simulink model "brake_in_car"  (R2024b)
settings: Solver=VariableStepAuto  StartTime=0.0  StopTime=inf  RelTol=1e-3
values from neighbouring files (symbols this model uses):
  A = 2    [evin_parameters.m]    (also in parameters.m)
  c_1 = 0.86    [evin_parameters.m]    (also in parameters.m)
  c_2 = 33.82    [evin_parameters.m]    (also in parameters.m)
  c_3 = 0.36    [evin_parameters.m]    (also in parameters.m)
  cw = 0.3    [parameters.m]
  g = 9.81    [evin_parameters.m]    (also in parameters.m)
  J = 0.8    [parameters.m]
  m = 1500    [evin_parameters.m]    (also in parameters.m)
  r = 0.3    [parameters.m]
  rho = 1.2    [evin_parameters.m]    (also in parameters.m)
  T_w = 5355    [parameters.m]
  x1 = 0    [parameters.m]
  x2 = 100    [parameters.m]
libraries: simulink x2
settings Model: Creator=kavin  LastModifiedBy=kavin
settings SolverCC: ZeroCrossAlgorithm=Adaptive
settings DebuggingCC: IgnoredZcDiagnostic=none

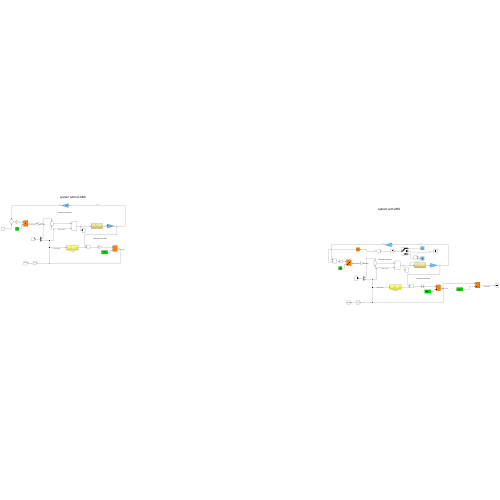
[thumbnail: Simulink's stored preview of the top-level diagram]
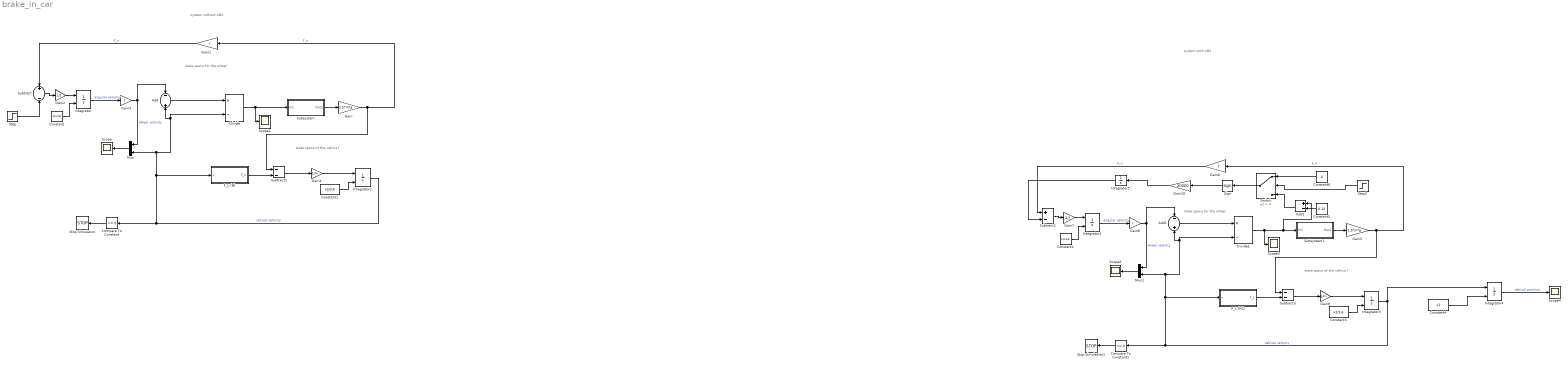
== system brake_in_car ==
  note: system without ABS
  note: state space of the vehica l
  note: state space for the wheel
  note: state space for the wheel
  note: state space of the vehica l
  note: system with ABS
  Add : Sum  Inputs=-+
  Add1 : Sum  Inputs=-+
  Add2 : Sum  Inputs=+-
  Compare To Constant : simulink/Logic and Bit Operations/Compare To Constant  relop=<=  const=0  OutDataTypeStr=boolean
  Compare To Constant1 : simulink/Logic and Bit Operations/Compare To Constant  relop=<=  const=0  OutDataTypeStr=boolean
  Constant : Constant  Value=x2/(r*3)
  Constant1 : Constant  Value=x2/3.6
  Constant2 : Constant  Value=x2/r/3.6
  Constant3 : Constant  Value=x2/3.6
  Constant4 : Constant  Value=x1
  Constant5 : Constant  Value=0.13
  Constant6 : Constant  Value=0
  Divide : Product  Inputs=*/
  Divide1 : Product  Inputs=*/
  F_L (N) : Subsystem
  F_L (N)1 : Subsystem
  Gain : Gain  Gain=1.5*m*g
  Gain{1,3,6,8} (4 alike) : Gain  Gain=r
  Gain10 : Gain  Gain=20000
  Gain2 : Gain  Gain=1/J
  Gain4 : Gain  Gain=1/m
  Gain5 : Gain  Gain=1.5*m*g
  Gain7 : Gain  Gain=1/J
  Gain9 : Gain  Gain=1/m
  Integrator : Integrator  InitialConditionSource=external
  Integrator1 : Integrator  InitialConditionSource=external  LimitOutput=on  LowerSaturationLimit=0
  Integrator2 : Integrator  InitialConditionSource=external
  Integrator3 : Integrator  InitialConditionSource=external  LimitOutput=on  LowerSaturationLimit=0
  Integrator4 : Integrator  InitialConditionSource=external  LimitOutput=on  LowerSaturationLimit=0
  Integrator5 : Integrator  LimitOutput=on  LowerSaturationLimit=0
  Mux : Mux  Inputs=2
  Mux1 : Mux  Inputs=2
  Scope{,1..4} (5 alike) : Scope
  Sign : Signum
  Step : Step  After=T_w  SampleTime=0
  Step2 : Step  SampleTime=0
  Stop Simulation : Stop
  Stop Simulation1 : Stop
  Subsystem : Subsystem
  Subsystem1 : Subsystem
  Subtract : Sum  Inputs=+-
  Subtract1 : Sum  Inputs=--
  Subtract2 : Sum  Inputs=+-
  Subtract3 : Sum  Inputs=--
  Switch : Switch  Criteria=u2 > Threshold  SaturateOnIntegerOverflow=off  InputSameDT=off
  wires:
  Subsystem/1(Out1) -> Gain/1
  Gain/1 -> Gain1/1, Subtract1/1  "F_n"
  Gain1/1 -> Subtract/1  "F_n"
  Step/1 -> Subtract/2
  Gain2/1 -> Integrator/1
  Subtract/1 -> Gain2/1
  Constant/1 -> Integrator/2
  Integrator/1 -> Gain3/1  "angular velocity"
  Gain3/1 -> Mux/1, Add/1  "wheel velocity"
  F_L (N)/1(F_L) -> Subtract1/2
  Subtract1/1 -> Gain4/1
  Gain4/1 -> Integrator2/1
  Integrator2/1 -> Compare To Constant/1, Divide/2, Add/2, Mux/2, F_L (N)/1(v)  "vehical velocity"
  Constant1/1 -> Integrator2/2
  Compare To Constant/1 -> Stop Simulation/1
  Mux/1 -> Scope/1
  Add/1 -> Divide/1
  Divide/1 -> Scope1/1, Subsystem/1(In1)
  Divide1/1 -> Scope3/1, Add2/2, Subsystem1/1(In1)
  Add1/1 -> Divide1/1
  Subtract2/1 -> Gain7/1
  Gain9/1 -> Integrator3/1
  Gain7/1 -> Integrator1/1
  Constant2/1 -> Integrator1/2
  Compare To Constant1/1 -> Stop Simulation1/1
  F_L (N)1/1(F_L) -> Subtract3/2
  Gain8/1 -> Mux1/1, Add1/1  "wheel velocity"
  Subtract3/1 -> Gain9/1
  Gain6/1 -> Subtract2/1  "F_n"
  Integrator3/1 -> Compare To Constant1/1, Divide1/2, Add1/2, Mux1/2, F_L (N)1/1(v), Integrator4/1  "vehical velocity"
  Subsystem1/1(Out1) -> Gain5/1
  Integrator1/1 -> Gain8/1  "angular velocity"
  Gain5/1 -> Gain6/1, Subtract3/1  "F_n"
  Mux1/1 -> Scope2/1
  Constant3/1 -> Integrator3/2
  Constant4/1 -> Integrator4/2
  Integrator4/1 -> Scope4/1  "vehical position"
  Add2/1 -> Switch/3
  Constant5/1 -> Add2/1
  Step2/1 -> Switch/2
  Switch/1 -> Sign/1
  Constant6/1 -> Switch/1
  Sign/1 -> Gain10/1
  Gain10/1 -> Integrator5/1
  Integrator5/1 -> Subtract2/2

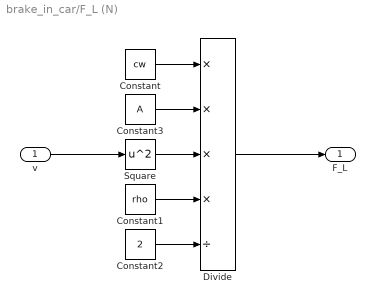
== system brake_in_car/F_L (N) ==
  v : Inport
  Constant : Constant  Value=cw
  Constant1 : Constant  Value=rho
  Constant2 : Constant  Value=2
  Constant3 : Constant  Value=A
  Divide : Product  Inputs=****/
  Square : Math  Operator=square
  F_L : Outport
  wires:
  v/1 -> Square/1
  Divide/1 -> F_L/1
  Square/1 -> Divide/3
  Constant2/1 -> Divide/5
  Constant/1 -> Divide/1
  Constant3/1 -> Divide/2
  Constant1/1 -> Divide/4

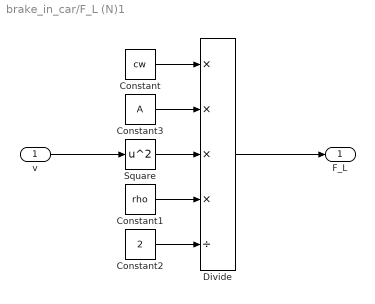
== system brake_in_car/F_L (N)1 ==
  v : Inport
  Constant : Constant  Value=cw
  Constant1 : Constant  Value=rho
  Constant2 : Constant  Value=2
  Constant3 : Constant  Value=A
  Divide : Product  Inputs=****/
  Square : Math  Operator=square
  F_L : Outport
  wires:
  v/1 -> Square/1
  Divide/1 -> F_L/1
  Square/1 -> Divide/3
  Constant2/1 -> Divide/5
  Constant/1 -> Divide/1
  Constant3/1 -> Divide/2
  Constant1/1 -> Divide/4

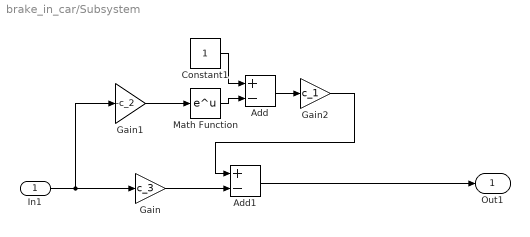
== system brake_in_car/Subsystem ==
  In1 : Inport
      settings: AttributesFormatString=|
      | %<BlockType>
      | lambda
  Add : Sum  Inputs=+-
  Add1 : Sum  Inputs=+-
  Constant1 : Constant
  Gain : Gain  Gain=c_3
  Gain1 : Gain  Gain=-c_2
  Gain2 : Gain  Gain=c_1
  Math Function : Math
  Out1 : Outport
      settings: AttributesFormatString=mu
  wires:
  In1/1 -> Gain1/1, Gain/1
  Gain1/1 -> Math Function/1
  Math Function/1 -> Add/2
  Constant1/1 -> Add/1
  Add/1 -> Gain2/1
  Gain2/1 -> Add1/1
  Add1/1 -> Out1/1
  Gain/1 -> Add1/2

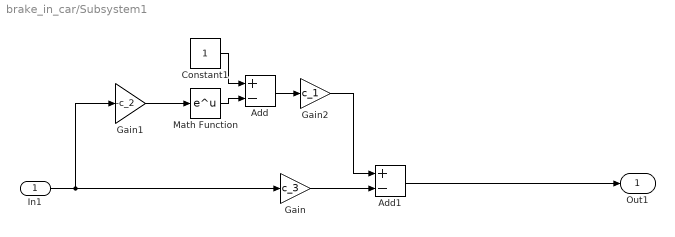
== system brake_in_car/Subsystem1 ==
  In1 : Inport
      settings: AttributesFormatString=|
      | %<BlockType>
      | lambda
  Add : Sum  Inputs=+-
  Add1 : Sum  Inputs=+-
  Constant1 : Constant
  Gain : Gain  Gain=c_3
  Gain1 : Gain  Gain=-c_2
  Gain2 : Gain  Gain=c_1
  Math Function : Math
  Out1 : Outport
      settings: AttributesFormatString=mu
  wires:
  In1/1 -> Gain1/1, Gain/1
  Gain1/1 -> Math Function/1
  Math Function/1 -> Add/2
  Constant1/1 -> Add/1
  Add/1 -> Gain2/1
  Gain2/1 -> Add1/1
  Add1/1 -> Out1/1
  Gain/1 -> Add1/2
